simulink model "TST_WESDem_CalcState"  (R2016b)
settings: Solver=FixedStepDiscrete  StartTime=0.0  StopTime=simTime  FixedStep=sampleTime  RelTol=1e-3
values from neighbouring files (symbols this model uses):
  testCase = 1    [initTST_WESDem_CalcState_001.m]    (also in initTST_WESDem_CalcState_002.m = 2; initTST_WESDem_CalcState_003.m = 3)
libraries: simulink x25, UnitTest_Lib x21
(part 2 of 2)

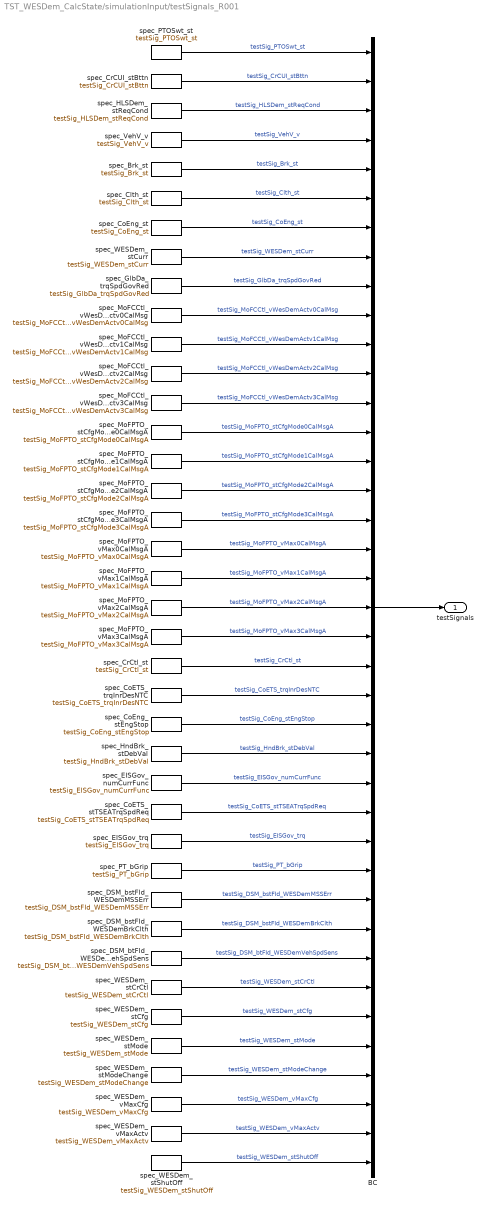
== system TST_WESDem_CalcState/simulationInput/testSignals_R001 ==
  BC : BusCreator  Inputs=39
  spec_Brk_st : FromWorkspace  VariableName=testSig_Brk_st  Interpolate=off  OutputAfterFinalValue=Holding final value
  spec_Clth_st : FromWorkspace  VariableName=testSig_Clth_st  Interpolate=off  OutputAfterFinalValue=Holding final value
  spec_CoETS_stTSEATrqSpdReq : FromWorkspace  VariableName=testSig_CoETS_stTSEATrqSpdReq  Interpolate=off  OutputAfterFinalValue=Holding final value
  spec_CoETS_trqInrDesNTC : FromWorkspace  VariableName=testSig_CoETS_trqInrDesNTC  Interpolate=off  OutputAfterFinalValue=Holding final value
  spec_CoEng_st : FromWorkspace  VariableName=testSig_CoEng_st  Interpolate=off  OutputAfterFinalValue=Holding final value
  spec_CoEng_stEngStop : FromWorkspace  VariableName=testSig_CoEng_stEngStop  Interpolate=off  OutputAfterFinalValue=Holding final value
  spec_CrCUI_stBttn : FromWorkspace  VariableName=testSig_CrCUI_stBttn  Interpolate=off  OutputAfterFinalValue=Holding final value
  spec_CrCtl_st : FromWorkspace  VariableName=testSig_CrCtl_st  Interpolate=off  OutputAfterFinalValue=Holding final value
  spec_DSM_bstFId_WESDemBrkClth : FromWorkspace  VariableName=testSig_DSM_bstFId_WESDemBrkClth  Interpolate=off  OutputAfterFinalValue=Holding final value
  spec_DSM_bstFId_WESDemMSSErr : FromWorkspace  VariableName=testSig_DSM_bstFId_WESDemMSSErr  Interpolate=off  OutputAfterFinalValue=Holding final value
  spec_DSM_btFId_WESDemVehSpdSens : FromWorkspace  VariableName=testSig_DSM_btFId_WESDemVehSpdSens  Interpolate=off  OutputAfterFinalValue=Holding final value
  spec_EISGov_numCurrFunc : FromWorkspace  VariableName=testSig_EISGov_numCurrFunc  Interpolate=off  OutputAfterFinalValue=Holding final value
  spec_EISGov_trq : FromWorkspace  VariableName=testSig_EISGov_trq  Interpolate=off  OutputAfterFinalValue=Holding final value
  spec_GlbDa_trqSpdGovRed : FromWorkspace  VariableName=testSig_GlbDa_trqSpdGovRed  Interpolate=off  OutputAfterFinalValue=Holding final value
  spec_HLSDem_stReqCond : FromWorkspace  VariableName=testSig_HLSDem_stReqCond  Interpolate=off  OutputAfterFinalValue=Holding final value
  spec_HndBrk_stDebVal : FromWorkspace  VariableName=testSig_HndBrk_stDebVal  Interpolate=off  OutputAfterFinalValue=Holding final value
  spec_MoFCCtl_vWesDemActv0CalMsg : FromWorkspace  VariableName=testSig_MoFCCtl_vWesDemActv0CalMsg  Interpolate=off  OutputAfterFinalValue=Holding final value
  spec_MoFCCtl_vWesDemActv1CalMsg : FromWorkspace  VariableName=testSig_MoFCCtl_vWesDemActv1CalMsg  Interpolate=off  OutputAfterFinalValue=Holding final value
  spec_MoFCCtl_vWesDemActv2CalMsg : FromWorkspace  VariableName=testSig_MoFCCtl_vWesDemActv2CalMsg  Interpolate=off  OutputAfterFinalValue=Holding final value
  spec_MoFCCtl_vWesDemActv3CalMsg : FromWorkspace  VariableName=testSig_MoFCCtl_vWesDemActv3CalMsg  Interpolate=off  OutputAfterFinalValue=Holding final value
  spec_MoFPTO_stCfgMode0CalMsgA : FromWorkspace  VariableName=testSig_MoFPTO_stCfgMode0CalMsgA  Interpolate=off  OutputAfterFinalValue=Holding final value
  spec_MoFPTO_stCfgMode1CalMsgA : FromWorkspace  VariableName=testSig_MoFPTO_stCfgMode1CalMsgA  Interpolate=off  OutputAfterFinalValue=Holding final value
  spec_MoFPTO_stCfgMode2CalMsgA : FromWorkspace  VariableName=testSig_MoFPTO_stCfgMode2CalMsgA  Interpolate=off  OutputAfterFinalValue=Holding final value
  spec_MoFPTO_stCfgMode3CalMsgA : FromWorkspace  VariableName=testSig_MoFPTO_stCfgMode3CalMsgA  Interpolate=off  OutputAfterFinalValue=Holding final value
  spec_MoFPTO_vMax0CalMsgA : FromWorkspace  VariableName=testSig_MoFPTO_vMax0CalMsgA  Interpolate=off  OutputAfterFinalValue=Holding final value
  spec_MoFPTO_vMax1CalMsgA : FromWorkspace  VariableName=testSig_MoFPTO_vMax1CalMsgA  Interpolate=off  OutputAfterFinalValue=Holding final value
  spec_MoFPTO_vMax2CalMsgA : FromWorkspace  VariableName=testSig_MoFPTO_vMax2CalMsgA  Interpolate=off  OutputAfterFinalValue=Holding final value
  spec_MoFPTO_vMax3CalMsgA : FromWorkspace  VariableName=testSig_MoFPTO_vMax3CalMsgA  Interpolate=off  OutputAfterFinalValue=Holding final value
  spec_PTOSwt_st : FromWorkspace  VariableName=testSig_PTOSwt_st  Interpolate=off  OutputAfterFinalValue=Holding final value
  spec_PT_bGrip : FromWorkspace  VariableName=testSig_PT_bGrip  Interpolate=off  OutputAfterFinalValue=Holding final value
  spec_VehV_v : FromWorkspace  VariableName=testSig_VehV_v  Interpolate=off  OutputAfterFinalValue=Holding final value
  spec_WESDem_stCfg : FromWorkspace  VariableName=testSig_WESDem_stCfg  Interpolate=off  OutputAfterFinalValue=Holding final value
  spec_WESDem_stCrCtl : FromWorkspace  VariableName=testSig_WESDem_stCrCtl  Interpolate=off  OutputAfterFinalValue=Holding final value
  spec_WESDem_stCurr : FromWorkspace  VariableName=testSig_WESDem_stCurr  Interpolate=off  OutputAfterFinalValue=Holding final value
  spec_WESDem_stMode : FromWorkspace  VariableName=testSig_WESDem_stMode  Interpolate=off  OutputAfterFinalValue=Holding final value
  spec_WESDem_stModeChange : FromWorkspace  VariableName=testSig_WESDem_stModeChange  Interpolate=off  OutputAfterFinalValue=Holding final value
  spec_WESDem_stShutOff : FromWorkspace  VariableName=testSig_WESDem_stShutOff  Interpolate=off  OutputAfterFinalValue=Holding final value
  spec_WESDem_vMaxActv : FromWorkspace  VariableName=testSig_WESDem_vMaxActv  Interpolate=off  OutputAfterFinalValue=Holding final value
  spec_WESDem_vMaxCfg : FromWorkspace  VariableName=testSig_WESDem_vMaxCfg  Interpolate=off  OutputAfterFinalValue=Holding final value
  testSignals : Outport
  wires:
  BC/1 -> testSignals/1
  spec_PTOSwt_st/1 -> BC/1  "testSig_PTOSwt_st"
  spec_CrCUI_stBttn/1 -> BC/2  "testSig_CrCUI_stBttn"
  spec_HLSDem_stReqCond/1 -> BC/3  "testSig_HLSDem_stReqCond"
  spec_VehV_v/1 -> BC/4  "testSig_VehV_v"
  spec_Brk_st/1 -> BC/5  "testSig_Brk_st"
  spec_Clth_st/1 -> BC/6  "testSig_Clth_st"
  spec_CoEng_st/1 -> BC/7  "testSig_CoEng_st"
  spec_WESDem_stCurr/1 -> BC/8  "testSig_WESDem_stCurr"
  spec_GlbDa_trqSpdGovRed/1 -> BC/9  "testSig_GlbDa_trqSpdGovRed"
  spec_MoFCCtl_vWesDemActv0CalMsg/1 -> BC/10  "testSig_MoFCCtl_vWesDemActv0CalMsg"
  spec_MoFCCtl_vWesDemActv1CalMsg/1 -> BC/11  "testSig_MoFCCtl_vWesDemActv1CalMsg"
  spec_MoFCCtl_vWesDemActv2CalMsg/1 -> BC/12  "testSig_MoFCCtl_vWesDemActv2CalMsg"
  spec_MoFCCtl_vWesDemActv3CalMsg/1 -> BC/13  "testSig_MoFCCtl_vWesDemActv3CalMsg"
  spec_MoFPTO_stCfgMode0CalMsgA/1 -> BC/14  "testSig_MoFPTO_stCfgMode0CalMsgA"
  spec_MoFPTO_stCfgMode1CalMsgA/1 -> BC/15  "testSig_MoFPTO_stCfgMode1CalMsgA"
  spec_MoFPTO_stCfgMode2CalMsgA/1 -> BC/16  "testSig_MoFPTO_stCfgMode2CalMsgA"
  spec_MoFPTO_stCfgMode3CalMsgA/1 -> BC/17  "testSig_MoFPTO_stCfgMode3CalMsgA"
  spec_MoFPTO_vMax0CalMsgA/1 -> BC/18  "testSig_MoFPTO_vMax0CalMsgA"
  spec_MoFPTO_vMax1CalMsgA/1 -> BC/19  "testSig_MoFPTO_vMax1CalMsgA"
  spec_MoFPTO_vMax2CalMsgA/1 -> BC/20  "testSig_MoFPTO_vMax2CalMsgA"
  spec_MoFPTO_vMax3CalMsgA/1 -> BC/21  "testSig_MoFPTO_vMax3CalMsgA"
  spec_CrCtl_st/1 -> BC/22  "testSig_CrCtl_st"
  spec_CoETS_trqInrDesNTC/1 -> BC/23  "testSig_CoETS_trqInrDesNTC"
  spec_CoEng_stEngStop/1 -> BC/24  "testSig_CoEng_stEngStop"
  spec_HndBrk_stDebVal/1 -> BC/25  "testSig_HndBrk_stDebVal"
  spec_EISGov_numCurrFunc/1 -> BC/26  "testSig_EISGov_numCurrFunc"
  spec_CoETS_stTSEATrqSpdReq/1 -> BC/27  "testSig_CoETS_stTSEATrqSpdReq"
  spec_EISGov_trq/1 -> BC/28  "testSig_EISGov_trq"
  spec_PT_bGrip/1 -> BC/29  "testSig_PT_bGrip"
  spec_DSM_bstFId_WESDemMSSErr/1 -> BC/30  "testSig_DSM_bstFId_WESDemMSSErr"
  spec_DSM_bstFId_WESDemBrkClth/1 -> BC/31  "testSig_DSM_bstFId_WESDemBrkClth"
  spec_DSM_btFId_WESDemVehSpdSens/1 -> BC/32  "testSig_DSM_btFId_WESDemVehSpdSens"
  spec_WESDem_stCrCtl/1 -> BC/33  "testSig_WESDem_stCrCtl"
  spec_WESDem_stCfg/1 -> BC/34  "testSig_WESDem_stCfg"
  spec_WESDem_stMode/1 -> BC/35  "testSig_WESDem_stMode"
  spec_WESDem_stModeChange/1 -> BC/36  "testSig_WESDem_stModeChange"
  spec_WESDem_vMaxCfg/1 -> BC/37  "testSig_WESDem_vMaxCfg"
  spec_WESDem_vMaxActv/1 -> BC/38  "testSig_WESDem_vMaxActv"
  spec_WESDem_stShutOff/1 -> BC/39  "testSig_WESDem_stShutOff"

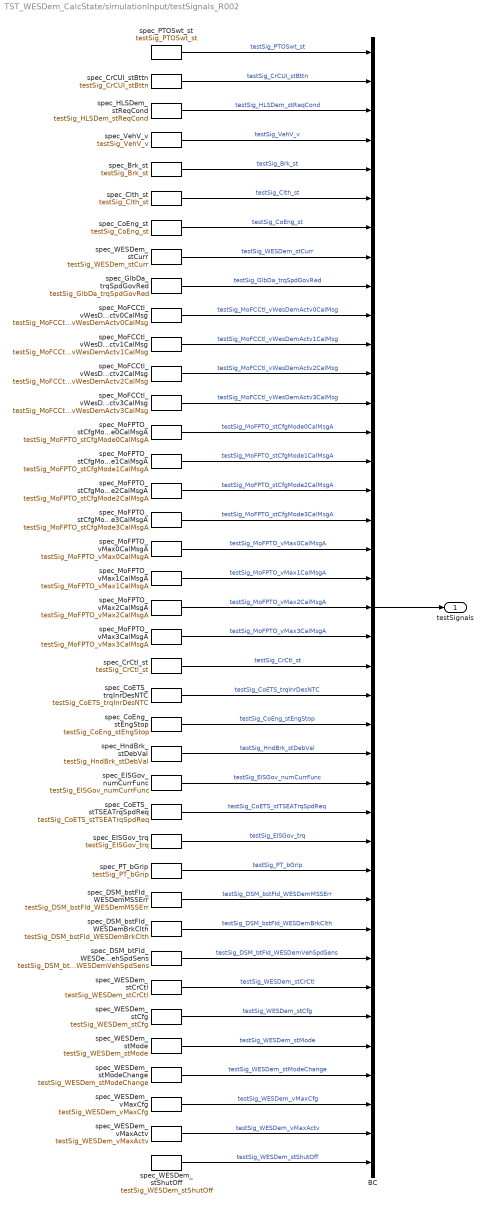
== system TST_WESDem_CalcState/simulationInput/testSignals_R002 ==
  BC : BusCreator  Inputs=39
  spec_Brk_st : FromWorkspace  VariableName=testSig_Brk_st  Interpolate=off  OutputAfterFinalValue=Holding final value
  spec_Clth_st : FromWorkspace  VariableName=testSig_Clth_st  Interpolate=off  OutputAfterFinalValue=Holding final value
  spec_CoETS_stTSEATrqSpdReq : FromWorkspace  VariableName=testSig_CoETS_stTSEATrqSpdReq  Interpolate=off  OutputAfterFinalValue=Holding final value
  spec_CoETS_trqInrDesNTC : FromWorkspace  VariableName=testSig_CoETS_trqInrDesNTC  Interpolate=off  OutputAfterFinalValue=Holding final value
  spec_CoEng_st : FromWorkspace  VariableName=testSig_CoEng_st  Interpolate=off  OutputAfterFinalValue=Holding final value
  spec_CoEng_stEngStop : FromWorkspace  VariableName=testSig_CoEng_stEngStop  Interpolate=off  OutputAfterFinalValue=Holding final value
  spec_CrCUI_stBttn : FromWorkspace  VariableName=testSig_CrCUI_stBttn  Interpolate=off  OutputAfterFinalValue=Holding final value
  spec_CrCtl_st : FromWorkspace  VariableName=testSig_CrCtl_st  Interpolate=off  OutputAfterFinalValue=Holding final value
  spec_DSM_bstFId_WESDemBrkClth : FromWorkspace  VariableName=testSig_DSM_bstFId_WESDemBrkClth  Interpolate=off  OutputAfterFinalValue=Holding final value
  spec_DSM_bstFId_WESDemMSSErr : FromWorkspace  VariableName=testSig_DSM_bstFId_WESDemMSSErr  Interpolate=off  OutputAfterFinalValue=Holding final value
  spec_DSM_btFId_WESDemVehSpdSens : FromWorkspace  VariableName=testSig_DSM_btFId_WESDemVehSpdSens  Interpolate=off  OutputAfterFinalValue=Holding final value
  spec_EISGov_numCurrFunc : FromWorkspace  VariableName=testSig_EISGov_numCurrFunc  Interpolate=off  OutputAfterFinalValue=Holding final value
  spec_EISGov_trq : FromWorkspace  VariableName=testSig_EISGov_trq  Interpolate=off  OutputAfterFinalValue=Holding final value
  spec_GlbDa_trqSpdGovRed : FromWorkspace  VariableName=testSig_GlbDa_trqSpdGovRed  Interpolate=off  OutputAfterFinalValue=Holding final value
  spec_HLSDem_stReqCond : FromWorkspace  VariableName=testSig_HLSDem_stReqCond  Interpolate=off  OutputAfterFinalValue=Holding final value
  spec_HndBrk_stDebVal : FromWorkspace  VariableName=testSig_HndBrk_stDebVal  Interpolate=off  OutputAfterFinalValue=Holding final value
  spec_MoFCCtl_vWesDemActv0CalMsg : FromWorkspace  VariableName=testSig_MoFCCtl_vWesDemActv0CalMsg  Interpolate=off  OutputAfterFinalValue=Holding final value
  spec_MoFCCtl_vWesDemActv1CalMsg : FromWorkspace  VariableName=testSig_MoFCCtl_vWesDemActv1CalMsg  Interpolate=off  OutputAfterFinalValue=Holding final value
  spec_MoFCCtl_vWesDemActv2CalMsg : FromWorkspace  VariableName=testSig_MoFCCtl_vWesDemActv2CalMsg  Interpolate=off  OutputAfterFinalValue=Holding final value
  spec_MoFCCtl_vWesDemActv3CalMsg : FromWorkspace  VariableName=testSig_MoFCCtl_vWesDemActv3CalMsg  Interpolate=off  OutputAfterFinalValue=Holding final value
  spec_MoFPTO_stCfgMode0CalMsgA : FromWorkspace  VariableName=testSig_MoFPTO_stCfgMode0CalMsgA  Interpolate=off  OutputAfterFinalValue=Holding final value
  spec_MoFPTO_stCfgMode1CalMsgA : FromWorkspace  VariableName=testSig_MoFPTO_stCfgMode1CalMsgA  Interpolate=off  OutputAfterFinalValue=Holding final value
  spec_MoFPTO_stCfgMode2CalMsgA : FromWorkspace  VariableName=testSig_MoFPTO_stCfgMode2CalMsgA  Interpolate=off  OutputAfterFinalValue=Holding final value
  spec_MoFPTO_stCfgMode3CalMsgA : FromWorkspace  VariableName=testSig_MoFPTO_stCfgMode3CalMsgA  Interpolate=off  OutputAfterFinalValue=Holding final value
  spec_MoFPTO_vMax0CalMsgA : FromWorkspace  VariableName=testSig_MoFPTO_vMax0CalMsgA  Interpolate=off  OutputAfterFinalValue=Holding final value
  spec_MoFPTO_vMax1CalMsgA : FromWorkspace  VariableName=testSig_MoFPTO_vMax1CalMsgA  Interpolate=off  OutputAfterFinalValue=Holding final value
  spec_MoFPTO_vMax2CalMsgA : FromWorkspace  VariableName=testSig_MoFPTO_vMax2CalMsgA  Interpolate=off  OutputAfterFinalValue=Holding final value
  spec_MoFPTO_vMax3CalMsgA : FromWorkspace  VariableName=testSig_MoFPTO_vMax3CalMsgA  Interpolate=off  OutputAfterFinalValue=Holding final value
  spec_PTOSwt_st : FromWorkspace  VariableName=testSig_PTOSwt_st  Interpolate=off  OutputAfterFinalValue=Holding final value
  spec_PT_bGrip : FromWorkspace  VariableName=testSig_PT_bGrip  Interpolate=off  OutputAfterFinalValue=Holding final value
  spec_VehV_v : FromWorkspace  VariableName=testSig_VehV_v  Interpolate=off  OutputAfterFinalValue=Holding final value
  spec_WESDem_stCfg : FromWorkspace  VariableName=testSig_WESDem_stCfg  Interpolate=off  OutputAfterFinalValue=Holding final value
  spec_WESDem_stCrCtl : FromWorkspace  VariableName=testSig_WESDem_stCrCtl  Interpolate=off  OutputAfterFinalValue=Holding final value
  spec_WESDem_stCurr : FromWorkspace  VariableName=testSig_WESDem_stCurr  Interpolate=off  OutputAfterFinalValue=Holding final value
  spec_WESDem_stMode : FromWorkspace  VariableName=testSig_WESDem_stMode  Interpolate=off  OutputAfterFinalValue=Holding final value
  spec_WESDem_stModeChange : FromWorkspace  VariableName=testSig_WESDem_stModeChange  Interpolate=off  OutputAfterFinalValue=Holding final value
  spec_WESDem_stShutOff : FromWorkspace  VariableName=testSig_WESDem_stShutOff  Interpolate=off  OutputAfterFinalValue=Holding final value
  spec_WESDem_vMaxActv : FromWorkspace  VariableName=testSig_WESDem_vMaxActv  Interpolate=off  OutputAfterFinalValue=Holding final value
  spec_WESDem_vMaxCfg : FromWorkspace  VariableName=testSig_WESDem_vMaxCfg  Interpolate=off  OutputAfterFinalValue=Holding final value
  testSignals : Outport
  wires:
  BC/1 -> testSignals/1
  spec_PTOSwt_st/1 -> BC/1  "testSig_PTOSwt_st"
  spec_CrCUI_stBttn/1 -> BC/2  "testSig_CrCUI_stBttn"
  spec_HLSDem_stReqCond/1 -> BC/3  "testSig_HLSDem_stReqCond"
  spec_VehV_v/1 -> BC/4  "testSig_VehV_v"
  spec_Brk_st/1 -> BC/5  "testSig_Brk_st"
  spec_Clth_st/1 -> BC/6  "testSig_Clth_st"
  spec_CoEng_st/1 -> BC/7  "testSig_CoEng_st"
  spec_WESDem_stCurr/1 -> BC/8  "testSig_WESDem_stCurr"
  spec_GlbDa_trqSpdGovRed/1 -> BC/9  "testSig_GlbDa_trqSpdGovRed"
  spec_MoFCCtl_vWesDemActv0CalMsg/1 -> BC/10  "testSig_MoFCCtl_vWesDemActv0CalMsg"
  spec_MoFCCtl_vWesDemActv1CalMsg/1 -> BC/11  "testSig_MoFCCtl_vWesDemActv1CalMsg"
  spec_MoFCCtl_vWesDemActv2CalMsg/1 -> BC/12  "testSig_MoFCCtl_vWesDemActv2CalMsg"
  spec_MoFCCtl_vWesDemActv3CalMsg/1 -> BC/13  "testSig_MoFCCtl_vWesDemActv3CalMsg"
  spec_MoFPTO_stCfgMode0CalMsgA/1 -> BC/14  "testSig_MoFPTO_stCfgMode0CalMsgA"
  spec_MoFPTO_stCfgMode1CalMsgA/1 -> BC/15  "testSig_MoFPTO_stCfgMode1CalMsgA"
  spec_MoFPTO_stCfgMode2CalMsgA/1 -> BC/16  "testSig_MoFPTO_stCfgMode2CalMsgA"
  spec_MoFPTO_stCfgMode3CalMsgA/1 -> BC/17  "testSig_MoFPTO_stCfgMode3CalMsgA"
  spec_MoFPTO_vMax0CalMsgA/1 -> BC/18  "testSig_MoFPTO_vMax0CalMsgA"
  spec_MoFPTO_vMax1CalMsgA/1 -> BC/19  "testSig_MoFPTO_vMax1CalMsgA"
  spec_MoFPTO_vMax2CalMsgA/1 -> BC/20  "testSig_MoFPTO_vMax2CalMsgA"
  spec_MoFPTO_vMax3CalMsgA/1 -> BC/21  "testSig_MoFPTO_vMax3CalMsgA"
  spec_CrCtl_st/1 -> BC/22  "testSig_CrCtl_st"
  spec_CoETS_trqInrDesNTC/1 -> BC/23  "testSig_CoETS_trqInrDesNTC"
  spec_CoEng_stEngStop/1 -> BC/24  "testSig_CoEng_stEngStop"
  spec_HndBrk_stDebVal/1 -> BC/25  "testSig_HndBrk_stDebVal"
  spec_EISGov_numCurrFunc/1 -> BC/26  "testSig_EISGov_numCurrFunc"
  spec_CoETS_stTSEATrqSpdReq/1 -> BC/27  "testSig_CoETS_stTSEATrqSpdReq"
  spec_EISGov_trq/1 -> BC/28  "testSig_EISGov_trq"
  spec_PT_bGrip/1 -> BC/29  "testSig_PT_bGrip"
  spec_DSM_bstFId_WESDemMSSErr/1 -> BC/30  "testSig_DSM_bstFId_WESDemMSSErr"
  spec_DSM_bstFId_WESDemBrkClth/1 -> BC/31  "testSig_DSM_bstFId_WESDemBrkClth"
  spec_DSM_btFId_WESDemVehSpdSens/1 -> BC/32  "testSig_DSM_btFId_WESDemVehSpdSens"
  spec_WESDem_stCrCtl/1 -> BC/33  "testSig_WESDem_stCrCtl"
  spec_WESDem_stCfg/1 -> BC/34  "testSig_WESDem_stCfg"
  spec_WESDem_stMode/1 -> BC/35  "testSig_WESDem_stMode"
  spec_WESDem_stModeChange/1 -> BC/36  "testSig_WESDem_stModeChange"
  spec_WESDem_vMaxCfg/1 -> BC/37  "testSig_WESDem_vMaxCfg"
  spec_WESDem_vMaxActv/1 -> BC/38  "testSig_WESDem_vMaxActv"
  spec_WESDem_stShutOff/1 -> BC/39  "testSig_WESDem_stShutOff"

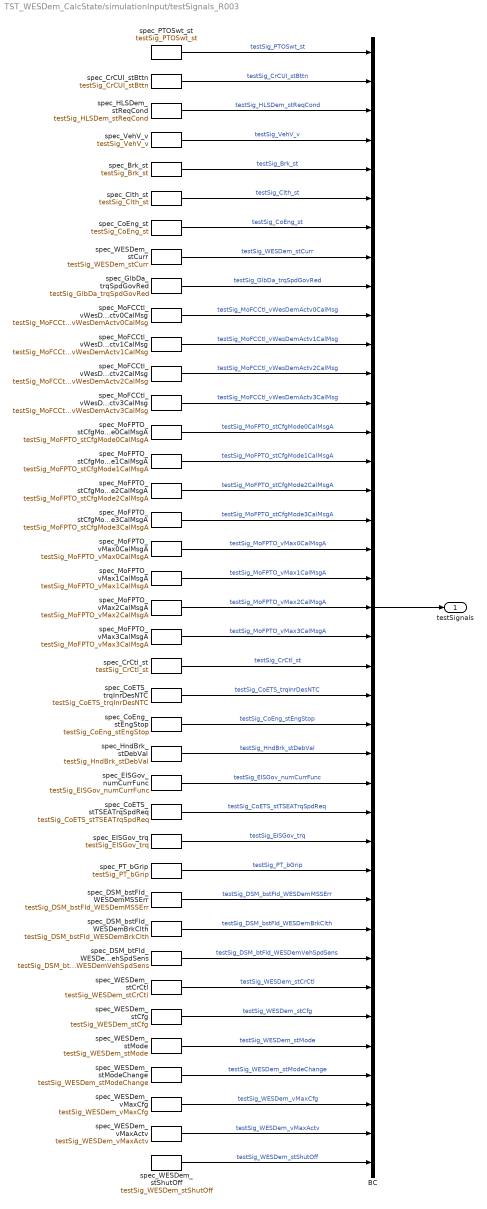
== system TST_WESDem_CalcState/simulationInput/testSignals_R003 ==
  BC : BusCreator  Inputs=39
  spec_Brk_st : FromWorkspace  VariableName=testSig_Brk_st  Interpolate=off  OutputAfterFinalValue=Holding final value
  spec_Clth_st : FromWorkspace  VariableName=testSig_Clth_st  Interpolate=off  OutputAfterFinalValue=Holding final value
  spec_CoETS_stTSEATrqSpdReq : FromWorkspace  VariableName=testSig_CoETS_stTSEATrqSpdReq  Interpolate=off  OutputAfterFinalValue=Holding final value
  spec_CoETS_trqInrDesNTC : FromWorkspace  VariableName=testSig_CoETS_trqInrDesNTC  Interpolate=off  OutputAfterFinalValue=Holding final value
  spec_CoEng_st : FromWorkspace  VariableName=testSig_CoEng_st  Interpolate=off  OutputAfterFinalValue=Holding final value
  spec_CoEng_stEngStop : FromWorkspace  VariableName=testSig_CoEng_stEngStop  Interpolate=off  OutputAfterFinalValue=Holding final value
  spec_CrCUI_stBttn : FromWorkspace  VariableName=testSig_CrCUI_stBttn  Interpolate=off  OutputAfterFinalValue=Holding final value
  spec_CrCtl_st : FromWorkspace  VariableName=testSig_CrCtl_st  Interpolate=off  OutputAfterFinalValue=Holding final value
  spec_DSM_bstFId_WESDemBrkClth : FromWorkspace  VariableName=testSig_DSM_bstFId_WESDemBrkClth  Interpolate=off  OutputAfterFinalValue=Holding final value
  spec_DSM_bstFId_WESDemMSSErr : FromWorkspace  VariableName=testSig_DSM_bstFId_WESDemMSSErr  Interpolate=off  OutputAfterFinalValue=Holding final value
  spec_DSM_btFId_WESDemVehSpdSens : FromWorkspace  VariableName=testSig_DSM_btFId_WESDemVehSpdSens  Interpolate=off  OutputAfterFinalValue=Holding final value
  spec_EISGov_numCurrFunc : FromWorkspace  VariableName=testSig_EISGov_numCurrFunc  Interpolate=off  OutputAfterFinalValue=Holding final value
  spec_EISGov_trq : FromWorkspace  VariableName=testSig_EISGov_trq  Interpolate=off  OutputAfterFinalValue=Holding final value
  spec_GlbDa_trqSpdGovRed : FromWorkspace  VariableName=testSig_GlbDa_trqSpdGovRed  Interpolate=off  OutputAfterFinalValue=Holding final value
  spec_HLSDem_stReqCond : FromWorkspace  VariableName=testSig_HLSDem_stReqCond  Interpolate=off  OutputAfterFinalValue=Holding final value
  spec_HndBrk_stDebVal : FromWorkspace  VariableName=testSig_HndBrk_stDebVal  Interpolate=off  OutputAfterFinalValue=Holding final value
  spec_MoFCCtl_vWesDemActv0CalMsg : FromWorkspace  VariableName=testSig_MoFCCtl_vWesDemActv0CalMsg  Interpolate=off  OutputAfterFinalValue=Holding final value
  spec_MoFCCtl_vWesDemActv1CalMsg : FromWorkspace  VariableName=testSig_MoFCCtl_vWesDemActv1CalMsg  Interpolate=off  OutputAfterFinalValue=Holding final value
  spec_MoFCCtl_vWesDemActv2CalMsg : FromWorkspace  VariableName=testSig_MoFCCtl_vWesDemActv2CalMsg  Interpolate=off  OutputAfterFinalValue=Holding final value
  spec_MoFCCtl_vWesDemActv3CalMsg : FromWorkspace  VariableName=testSig_MoFCCtl_vWesDemActv3CalMsg  Interpolate=off  OutputAfterFinalValue=Holding final value
  spec_MoFPTO_stCfgMode0CalMsgA : FromWorkspace  VariableName=testSig_MoFPTO_stCfgMode0CalMsgA  Interpolate=off  OutputAfterFinalValue=Holding final value
  spec_MoFPTO_stCfgMode1CalMsgA : FromWorkspace  VariableName=testSig_MoFPTO_stCfgMode1CalMsgA  Interpolate=off  OutputAfterFinalValue=Holding final value
  spec_MoFPTO_stCfgMode2CalMsgA : FromWorkspace  VariableName=testSig_MoFPTO_stCfgMode2CalMsgA  Interpolate=off  OutputAfterFinalValue=Holding final value
  spec_MoFPTO_stCfgMode3CalMsgA : FromWorkspace  VariableName=testSig_MoFPTO_stCfgMode3CalMsgA  Interpolate=off  OutputAfterFinalValue=Holding final value
  spec_MoFPTO_vMax0CalMsgA : FromWorkspace  VariableName=testSig_MoFPTO_vMax0CalMsgA  Interpolate=off  OutputAfterFinalValue=Holding final value
  spec_MoFPTO_vMax1CalMsgA : FromWorkspace  VariableName=testSig_MoFPTO_vMax1CalMsgA  Interpolate=off  OutputAfterFinalValue=Holding final value
  spec_MoFPTO_vMax2CalMsgA : FromWorkspace  VariableName=testSig_MoFPTO_vMax2CalMsgA  Interpolate=off  OutputAfterFinalValue=Holding final value
  spec_MoFPTO_vMax3CalMsgA : FromWorkspace  VariableName=testSig_MoFPTO_vMax3CalMsgA  Interpolate=off  OutputAfterFinalValue=Holding final value
  spec_PTOSwt_st : FromWorkspace  VariableName=testSig_PTOSwt_st  Interpolate=off  OutputAfterFinalValue=Holding final value
  spec_PT_bGrip : FromWorkspace  VariableName=testSig_PT_bGrip  Interpolate=off  OutputAfterFinalValue=Holding final value
  spec_VehV_v : FromWorkspace  VariableName=testSig_VehV_v  Interpolate=off  OutputAfterFinalValue=Holding final value
  spec_WESDem_stCfg : FromWorkspace  VariableName=testSig_WESDem_stCfg  Interpolate=off  OutputAfterFinalValue=Holding final value
  spec_WESDem_stCrCtl : FromWorkspace  VariableName=testSig_WESDem_stCrCtl  Interpolate=off  OutputAfterFinalValue=Holding final value
  spec_WESDem_stCurr : FromWorkspace  VariableName=testSig_WESDem_stCurr  Interpolate=off  OutputAfterFinalValue=Holding final value
  spec_WESDem_stMode : FromWorkspace  VariableName=testSig_WESDem_stMode  Interpolate=off  OutputAfterFinalValue=Holding final value
  spec_WESDem_stModeChange : FromWorkspace  VariableName=testSig_WESDem_stModeChange  Interpolate=off  OutputAfterFinalValue=Holding final value
  spec_WESDem_stShutOff : FromWorkspace  VariableName=testSig_WESDem_stShutOff  Interpolate=off  OutputAfterFinalValue=Holding final value
  spec_WESDem_vMaxActv : FromWorkspace  VariableName=testSig_WESDem_vMaxActv  Interpolate=off  OutputAfterFinalValue=Holding final value
  spec_WESDem_vMaxCfg : FromWorkspace  VariableName=testSig_WESDem_vMaxCfg  Interpolate=off  OutputAfterFinalValue=Holding final value
  testSignals : Outport
  wires:
  BC/1 -> testSignals/1
  spec_PTOSwt_st/1 -> BC/1  "testSig_PTOSwt_st"
  spec_CrCUI_stBttn/1 -> BC/2  "testSig_CrCUI_stBttn"
  spec_HLSDem_stReqCond/1 -> BC/3  "testSig_HLSDem_stReqCond"
  spec_VehV_v/1 -> BC/4  "testSig_VehV_v"
  spec_Brk_st/1 -> BC/5  "testSig_Brk_st"
  spec_Clth_st/1 -> BC/6  "testSig_Clth_st"
  spec_CoEng_st/1 -> BC/7  "testSig_CoEng_st"
  spec_WESDem_stCurr/1 -> BC/8  "testSig_WESDem_stCurr"
  spec_GlbDa_trqSpdGovRed/1 -> BC/9  "testSig_GlbDa_trqSpdGovRed"
  spec_MoFCCtl_vWesDemActv0CalMsg/1 -> BC/10  "testSig_MoFCCtl_vWesDemActv0CalMsg"
  spec_MoFCCtl_vWesDemActv1CalMsg/1 -> BC/11  "testSig_MoFCCtl_vWesDemActv1CalMsg"
  spec_MoFCCtl_vWesDemActv2CalMsg/1 -> BC/12  "testSig_MoFCCtl_vWesDemActv2CalMsg"
  spec_MoFCCtl_vWesDemActv3CalMsg/1 -> BC/13  "testSig_MoFCCtl_vWesDemActv3CalMsg"
  spec_MoFPTO_stCfgMode0CalMsgA/1 -> BC/14  "testSig_MoFPTO_stCfgMode0CalMsgA"
  spec_MoFPTO_stCfgMode1CalMsgA/1 -> BC/15  "testSig_MoFPTO_stCfgMode1CalMsgA"
  spec_MoFPTO_stCfgMode2CalMsgA/1 -> BC/16  "testSig_MoFPTO_stCfgMode2CalMsgA"
  spec_MoFPTO_stCfgMode3CalMsgA/1 -> BC/17  "testSig_MoFPTO_stCfgMode3CalMsgA"
  spec_MoFPTO_vMax0CalMsgA/1 -> BC/18  "testSig_MoFPTO_vMax0CalMsgA"
  spec_MoFPTO_vMax1CalMsgA/1 -> BC/19  "testSig_MoFPTO_vMax1CalMsgA"
  spec_MoFPTO_vMax2CalMsgA/1 -> BC/20  "testSig_MoFPTO_vMax2CalMsgA"
  spec_MoFPTO_vMax3CalMsgA/1 -> BC/21  "testSig_MoFPTO_vMax3CalMsgA"
  spec_CrCtl_st/1 -> BC/22  "testSig_CrCtl_st"
  spec_CoETS_trqInrDesNTC/1 -> BC/23  "testSig_CoETS_trqInrDesNTC"
  spec_CoEng_stEngStop/1 -> BC/24  "testSig_CoEng_stEngStop"
  spec_HndBrk_stDebVal/1 -> BC/25  "testSig_HndBrk_stDebVal"
  spec_EISGov_numCurrFunc/1 -> BC/26  "testSig_EISGov_numCurrFunc"
  spec_CoETS_stTSEATrqSpdReq/1 -> BC/27  "testSig_CoETS_stTSEATrqSpdReq"
  spec_EISGov_trq/1 -> BC/28  "testSig_EISGov_trq"
  spec_PT_bGrip/1 -> BC/29  "testSig_PT_bGrip"
  spec_DSM_bstFId_WESDemMSSErr/1 -> BC/30  "testSig_DSM_bstFId_WESDemMSSErr"
  spec_DSM_bstFId_WESDemBrkClth/1 -> BC/31  "testSig_DSM_bstFId_WESDemBrkClth"
  spec_DSM_btFId_WESDemVehSpdSens/1 -> BC/32  "testSig_DSM_btFId_WESDemVehSpdSens"
  spec_WESDem_stCrCtl/1 -> BC/33  "testSig_WESDem_stCrCtl"
  spec_WESDem_stCfg/1 -> BC/34  "testSig_WESDem_stCfg"
  spec_WESDem_stMode/1 -> BC/35  "testSig_WESDem_stMode"
  spec_WESDem_stModeChange/1 -> BC/36  "testSig_WESDem_stModeChange"
  spec_WESDem_vMaxCfg/1 -> BC/37  "testSig_WESDem_vMaxCfg"
  spec_WESDem_vMaxActv/1 -> BC/38  "testSig_WESDem_vMaxActv"
  spec_WESDem_stShutOff/1 -> BC/39  "testSig_WESDem_stShutOff"

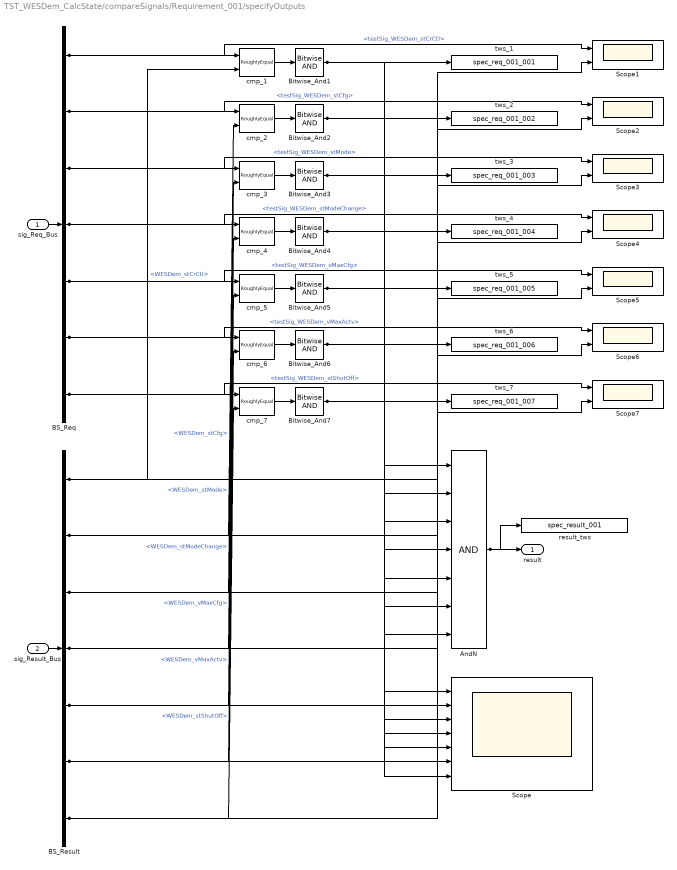
== system TST_WESDem_CalcState/compareSignals/Requirement_001/specifyOutputs ==
  sig_Req_Bus : Inport
  sig_Result_Bus : Inport  Port=2
  AndN : Logic  Inputs=7
  BS_Req : BusSelector  OutputSignals=testSig_WESDem_stCrCtl,testSig_WESDem_stCfg,testSig_WESDem_stMode,testSig_WESDem_stModeChange,testSig_WESDem_vMaxCfg,testSig_WESDem_vMaxActv,testSig_WESDem_stShutOff
  BS_Result : BusSelector  OutputSignals=WESDem_stCrCtl,WESDem_stCfg,WESDem_stMode,WESDem_stModeChange,WESDem_vMaxCfg,WESDem_vMaxActv,WESDem_stShutOff
  Bitwise_And{1..7} (7 alike) : simulink/Logic and Bit Operations/Bitwise Operator  logicop=AND  UseBitMask=off  BitMask=bin2dec('11011001')  BitMaskRealWorld=Stored Integer
  Scope : Scope  NumInputPorts=7
  Scope{1..7} (7 alike) : Scope  NumInputPorts=2
  cmp_{1..7} (7 alike) : UnitTest_Lib/RoughlyEqual  slope=0.1
  result_tws : ToWorkspace  VariableName=spec_result_001
  tws_1 : ToWorkspace  VariableName=spec_req_001_001
  tws_2 : ToWorkspace  VariableName=spec_req_001_002
  tws_3 : ToWorkspace  VariableName=spec_req_001_003
  tws_4 : ToWorkspace  VariableName=spec_req_001_004
  tws_5 : ToWorkspace  VariableName=spec_req_001_005
  tws_6 : ToWorkspace  VariableName=spec_req_001_006
  tws_7 : ToWorkspace  VariableName=spec_req_001_007
  result : Outport
  wires:
  sig_Req_Bus/1 -> BS_Req/1
  sig_Result_Bus/1 -> BS_Result/1
  AndN/1 -> result/1, result_tws/1
  BS_Req/1 -> cmp_1/1, Scope1/1  "<testSig_WESDem_stCrCtl>"
  BS_Result/1 -> cmp_1/2, Scope1/2  "<WESDem_stCrCtl>"
  cmp_1/1 -> Bitwise_And1/1
  Bitwise_And1/1 -> tws_1/1, AndN/1, Scope/1
  BS_Req/2 -> cmp_2/1, Scope2/1  "<testSig_WESDem_stCfg>"
  BS_Result/2 -> cmp_2/2, Scope2/2  "<WESDem_stCfg>"
  cmp_2/1 -> Bitwise_And2/1
  Bitwise_And2/1 -> tws_2/1, AndN/2, Scope/2
  BS_Req/3 -> cmp_3/1, Scope3/1  "<testSig_WESDem_stMode>"
  BS_Result/3 -> cmp_3/2, Scope3/2  "<WESDem_stMode>"
  cmp_3/1 -> Bitwise_And3/1
  Bitwise_And3/1 -> tws_3/1, AndN/3, Scope/3
  BS_Req/4 -> cmp_4/1, Scope4/1  "<testSig_WESDem_stModeChange>"
  BS_Result/4 -> cmp_4/2, Scope4/2  "<WESDem_stModeChange>"
  cmp_4/1 -> Bitwise_And4/1
  Bitwise_And4/1 -> tws_4/1, AndN/4, Scope/4
  BS_Req/5 -> cmp_5/1, Scope5/1  "<testSig_WESDem_vMaxCfg>"
  BS_Result/5 -> cmp_5/2, Scope5/2  "<WESDem_vMaxCfg>"
  cmp_5/1 -> Bitwise_And5/1
  Bitwise_And5/1 -> tws_5/1, AndN/5, Scope/5
  BS_Req/6 -> cmp_6/1, Scope6/1  "<testSig_WESDem_vMaxActv>"
  BS_Result/6 -> cmp_6/2, Scope6/2  "<WESDem_vMaxActv>"
  cmp_6/1 -> Bitwise_And6/1
  Bitwise_And6/1 -> tws_6/1, AndN/6, Scope/6
  BS_Req/7 -> cmp_7/1, Scope7/1  "<testSig_WESDem_stShutOff>"
  BS_Result/7 -> cmp_7/2, Scope7/2  "<WESDem_stShutOff>"
  cmp_7/1 -> Bitwise_And7/1
  Bitwise_And7/1 -> tws_7/1, AndN/7, Scope/7

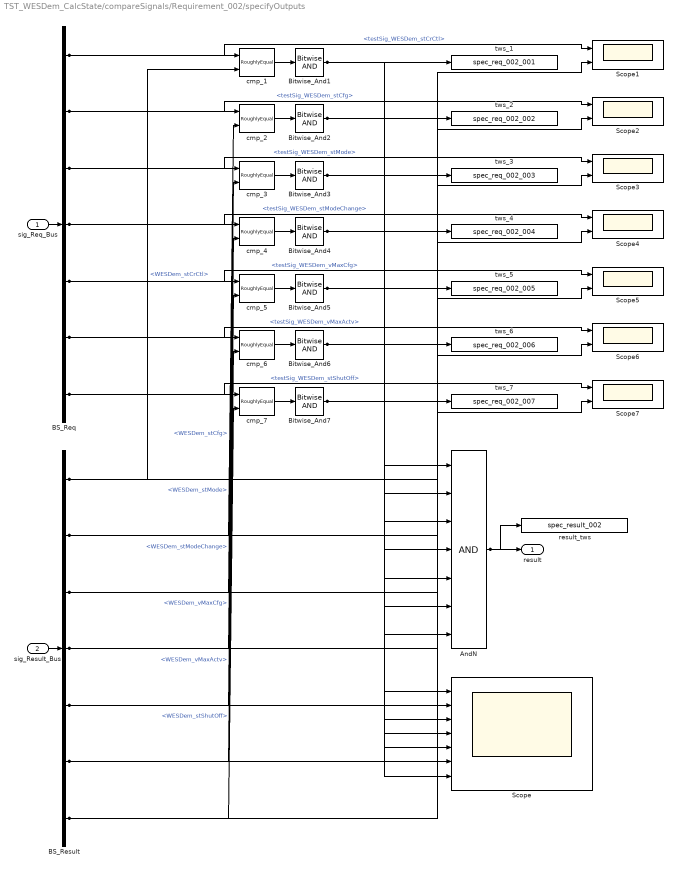
== system TST_WESDem_CalcState/compareSignals/Requirement_002/specifyOutputs ==
  sig_Req_Bus : Inport
  sig_Result_Bus : Inport  Port=2
  AndN : Logic  Inputs=7
  BS_Req : BusSelector  OutputSignals=testSig_WESDem_stCrCtl,testSig_WESDem_stCfg,testSig_WESDem_stMode,testSig_WESDem_stModeChange,testSig_WESDem_vMaxCfg,testSig_WESDem_vMaxActv,testSig_WESDem_stShutOff
  BS_Result : BusSelector  OutputSignals=WESDem_stCrCtl,WESDem_stCfg,WESDem_stMode,WESDem_stModeChange,WESDem_vMaxCfg,WESDem_vMaxActv,WESDem_stShutOff
  Bitwise_And{1..7} (7 alike) : simulink/Logic and Bit Operations/Bitwise Operator  logicop=AND  UseBitMask=off  BitMask=bin2dec('11011001')  BitMaskRealWorld=Stored Integer
  Scope : Scope  NumInputPorts=7
  Scope{1..7} (7 alike) : Scope  NumInputPorts=2
  cmp_{1..7} (7 alike) : UnitTest_Lib/RoughlyEqual  slope=0.1
  result_tws : ToWorkspace  VariableName=spec_result_002
  tws_1 : ToWorkspace  VariableName=spec_req_002_001
  tws_2 : ToWorkspace  VariableName=spec_req_002_002
  tws_3 : ToWorkspace  VariableName=spec_req_002_003
  tws_4 : ToWorkspace  VariableName=spec_req_002_004
  tws_5 : ToWorkspace  VariableName=spec_req_002_005
  tws_6 : ToWorkspace  VariableName=spec_req_002_006
  tws_7 : ToWorkspace  VariableName=spec_req_002_007
  result : Outport
  wires:
  sig_Req_Bus/1 -> BS_Req/1
  sig_Result_Bus/1 -> BS_Result/1
  AndN/1 -> result/1, result_tws/1
  BS_Req/1 -> cmp_1/1, Scope1/1  "<testSig_WESDem_stCrCtl>"
  BS_Result/1 -> cmp_1/2, Scope1/2  "<WESDem_stCrCtl>"
  cmp_1/1 -> Bitwise_And1/1
  Bitwise_And1/1 -> tws_1/1, AndN/1, Scope/1
  BS_Req/2 -> cmp_2/1, Scope2/1  "<testSig_WESDem_stCfg>"
  BS_Result/2 -> cmp_2/2, Scope2/2  "<WESDem_stCfg>"
  cmp_2/1 -> Bitwise_And2/1
  Bitwise_And2/1 -> tws_2/1, AndN/2, Scope/2
  BS_Req/3 -> cmp_3/1, Scope3/1  "<testSig_WESDem_stMode>"
  BS_Result/3 -> cmp_3/2, Scope3/2  "<WESDem_stMode>"
  cmp_3/1 -> Bitwise_And3/1
  Bitwise_And3/1 -> tws_3/1, AndN/3, Scope/3
  BS_Req/4 -> cmp_4/1, Scope4/1  "<testSig_WESDem_stModeChange>"
  BS_Result/4 -> cmp_4/2, Scope4/2  "<WESDem_stModeChange>"
  cmp_4/1 -> Bitwise_And4/1
  Bitwise_And4/1 -> tws_4/1, AndN/4, Scope/4
  BS_Req/5 -> cmp_5/1, Scope5/1  "<testSig_WESDem_vMaxCfg>"
  BS_Result/5 -> cmp_5/2, Scope5/2  "<WESDem_vMaxCfg>"
  cmp_5/1 -> Bitwise_And5/1
  Bitwise_And5/1 -> tws_5/1, AndN/5, Scope/5
  BS_Req/6 -> cmp_6/1, Scope6/1  "<testSig_WESDem_vMaxActv>"
  BS_Result/6 -> cmp_6/2, Scope6/2  "<WESDem_vMaxActv>"
  cmp_6/1 -> Bitwise_And6/1
  Bitwise_And6/1 -> tws_6/1, AndN/6, Scope/6
  BS_Req/7 -> cmp_7/1, Scope7/1  "<testSig_WESDem_stShutOff>"
  BS_Result/7 -> cmp_7/2, Scope7/2  "<WESDem_stShutOff>"
  cmp_7/1 -> Bitwise_And7/1
  Bitwise_And7/1 -> tws_7/1, AndN/7, Scope/7

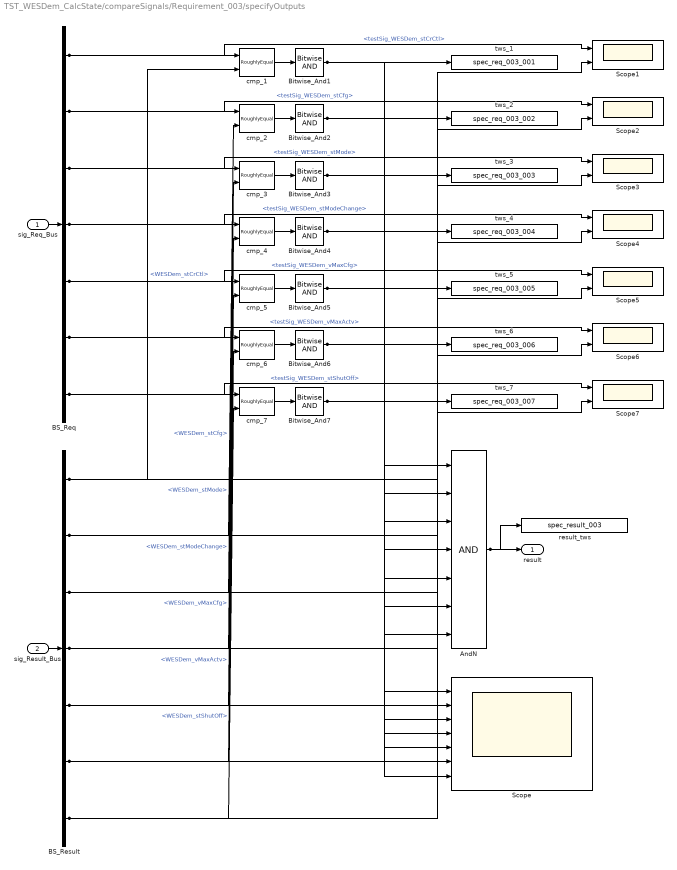
== system TST_WESDem_CalcState/compareSignals/Requirement_003/specifyOutputs ==
  sig_Req_Bus : Inport
  sig_Result_Bus : Inport  Port=2
  AndN : Logic  Inputs=7
  BS_Req : BusSelector  OutputSignals=testSig_WESDem_stCrCtl,testSig_WESDem_stCfg,testSig_WESDem_stMode,testSig_WESDem_stModeChange,testSig_WESDem_vMaxCfg,testSig_WESDem_vMaxActv,testSig_WESDem_stShutOff
  BS_Result : BusSelector  OutputSignals=WESDem_stCrCtl,WESDem_stCfg,WESDem_stMode,WESDem_stModeChange,WESDem_vMaxCfg,WESDem_vMaxActv,WESDem_stShutOff
  Bitwise_And{1..7} (7 alike) : simulink/Logic and Bit Operations/Bitwise Operator  logicop=AND  UseBitMask=off  BitMask=bin2dec('11011001')  BitMaskRealWorld=Stored Integer
  Scope : Scope  NumInputPorts=7
  Scope{1..7} (7 alike) : Scope  NumInputPorts=2
  cmp_{1..7} (7 alike) : UnitTest_Lib/RoughlyEqual  slope=0.1
  result_tws : ToWorkspace  VariableName=spec_result_003
  tws_1 : ToWorkspace  VariableName=spec_req_003_001
  tws_2 : ToWorkspace  VariableName=spec_req_003_002
  tws_3 : ToWorkspace  VariableName=spec_req_003_003
  tws_4 : ToWorkspace  VariableName=spec_req_003_004
  tws_5 : ToWorkspace  VariableName=spec_req_003_005
  tws_6 : ToWorkspace  VariableName=spec_req_003_006
  tws_7 : ToWorkspace  VariableName=spec_req_003_007
  result : Outport
  wires:
  sig_Req_Bus/1 -> BS_Req/1
  sig_Result_Bus/1 -> BS_Result/1
  AndN/1 -> result/1, result_tws/1
  BS_Req/1 -> cmp_1/1, Scope1/1  "<testSig_WESDem_stCrCtl>"
  BS_Result/1 -> cmp_1/2, Scope1/2  "<WESDem_stCrCtl>"
  cmp_1/1 -> Bitwise_And1/1
  Bitwise_And1/1 -> tws_1/1, AndN/1, Scope/1
  BS_Req/2 -> cmp_2/1, Scope2/1  "<testSig_WESDem_stCfg>"
  BS_Result/2 -> cmp_2/2, Scope2/2  "<WESDem_stCfg>"
  cmp_2/1 -> Bitwise_And2/1
  Bitwise_And2/1 -> tws_2/1, AndN/2, Scope/2
  BS_Req/3 -> cmp_3/1, Scope3/1  "<testSig_WESDem_stMode>"
  BS_Result/3 -> cmp_3/2, Scope3/2  "<WESDem_stMode>"
  cmp_3/1 -> Bitwise_And3/1
  Bitwise_And3/1 -> tws_3/1, AndN/3, Scope/3
  BS_Req/4 -> cmp_4/1, Scope4/1  "<testSig_WESDem_stModeChange>"
  BS_Result/4 -> cmp_4/2, Scope4/2  "<WESDem_stModeChange>"
  cmp_4/1 -> Bitwise_And4/1
  Bitwise_And4/1 -> tws_4/1, AndN/4, Scope/4
  BS_Req/5 -> cmp_5/1, Scope5/1  "<testSig_WESDem_vMaxCfg>"
  BS_Result/5 -> cmp_5/2, Scope5/2  "<WESDem_vMaxCfg>"
  cmp_5/1 -> Bitwise_And5/1
  Bitwise_And5/1 -> tws_5/1, AndN/5, Scope/5
  BS_Req/6 -> cmp_6/1, Scope6/1  "<testSig_WESDem_vMaxActv>"
  BS_Result/6 -> cmp_6/2, Scope6/2  "<WESDem_vMaxActv>"
  cmp_6/1 -> Bitwise_And6/1
  Bitwise_And6/1 -> tws_6/1, AndN/6, Scope/6
  BS_Req/7 -> cmp_7/1, Scope7/1  "<testSig_WESDem_stShutOff>"
  BS_Result/7 -> cmp_7/2, Scope7/2  "<WESDem_stShutOff>"
  cmp_7/1 -> Bitwise_And7/1
  Bitwise_And7/1 -> tws_7/1, AndN/7, Scope/7
